simulink model "sf_fitness"  (R2017b)
settings: Solver=FixedStepAuto  StartTime=0.0  StopTime=inf  FixedStep=0.001  RelTol=1e-3  EnableMultiTasking=on
StopFcn:
  | close all force;
  | set_param('sf_fitness/Stop', 'Value', '0');
undefined symbols (not defined in the file): ActivityType
settings Model: Creator=The MathWorks, Inc.  LastModifiedBy=The MathWorks, Inc.
settings SolverCC: IsAutoAppliedInSIP=on
settings DataIOCC: LimitDataPoints=on
settings OptimizationCC: LifeSpan=inf
settings DebuggingCC: AllowSymbolicDim=off  SFUnexpectedBacktrackingDiag=warning  SFNoUnconditionalDefaultTransitionDiag=warning  SFExecutionAtInitializationDiag=none
settings ModelReferenceCC: PropagateSignalLabelsOutOfModel=off
settings CodeAppCC: StateflowObjectComments=on
settings GRTTargetCC: TargetLangStandard=C89/C90 (ANSI)
settings ConfigComp: CovMetricSettings=dw  CovHtmlReporting=on  CovSaveCumulativeToWorkspaceVar=on  CovSaveSingleToWorkspaceVar=on  CovExternalEMLEnable=off
settings SimscapeCC: SimscapeNormalizeSystem=off  SimscapeNominalValues={1, 'bar'; 1, 'cm^3/s'; 1, 'bar*kg/s'; 1, 'kJ/kg'; 1, 'kW'}

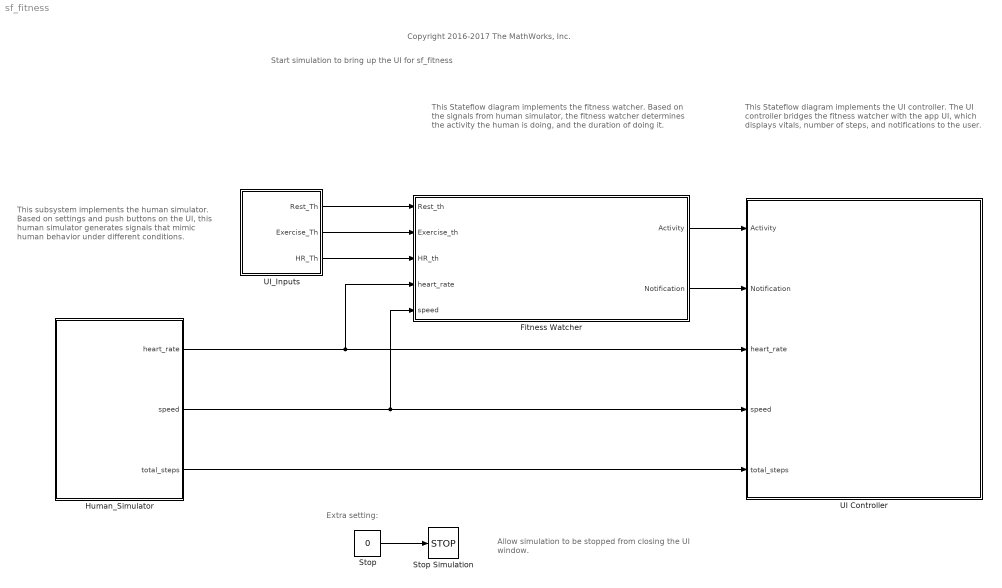
== system sf_fitness ==
  note: Extra setting:
  note: Allow simulation to be stopped from
      | closing the UI window.
  note: This subsystem implements
      | the human simulator.
      |
      | Based on settings and push buttons on
      | the UI, this human simulator generates
      | signals that mimic human behavior under
      | different conditions.
  note: This Stateflow diagram implements
      | the fitness watcher.
      |
      | Based on the signals from human simulator,
      | the fitness watcher determines the activity
      | the human is doing, and the duration of doing it.
  note: Start simulation to bring up the UI for sf_fitness
  note: This Stateflow diagram implements
      | the UI controller.
      |
      | The UI controller bridges the fitness watcher with the app UI, which displays vitals, number of steps, and notifications to the user.
  note: Copyright 2016-2017 The MathWorks, Inc.
  Fitness Watcher : Stateflow chart  TreatAsAtomicUnit=on
  Human_Simulator : Subsystem
  Stop : Constant  Value=0
  Stop Simulation : Stop
  UI Controller : Stateflow chart  TreatAsAtomicUnit=on
  UI_Inputs : Subsystem
  wires:
  Fitness Watcher/2(Notification) -> UI Controller/2(Notification)
  UI_Inputs/1(Rest_Th) -> Fitness Watcher/1(Rest_th)
  UI_Inputs/2(Exercise_Th) -> Fitness Watcher/2(Exercise_th)
  UI_Inputs/3(HR_Th) -> Fitness Watcher/3(HR_th)
  Fitness Watcher/1(Activity) -> UI Controller/1(Activity)
  Human_Simulator/1(heart_rate) -> Fitness Watcher/4(heart_rate), UI Controller/3(heart_rate)
  Human_Simulator/2(speed) -> Fitness Watcher/5(speed), UI Controller/4(speed)
  Human_Simulator/3(total_steps) -> UI Controller/5(total_steps)
  Stop/1 -> Stop Simulation/1

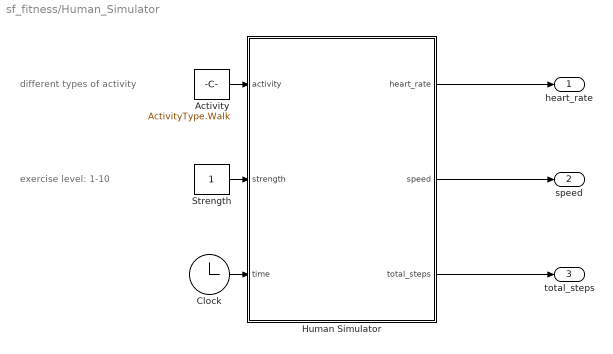
== system sf_fitness/Human_Simulator ==
  note: different types of activity
  note: exercise level: 1-10
  Activity : Constant  Value=ActivityType.Walk
  Clock : Clock
  Human Simulator : Stateflow chart  TreatAsAtomicUnit=on
  Strength : Constant
  heart_rate : Outport
  speed : Outport  Port=2
  total_steps : Outport  Port=3
  wires:
  Activity/1 -> Human Simulator/1(activity)
  Human Simulator/3(total_steps) -> total_steps/1
  Clock/1 -> Human Simulator/3(time)
  Strength/1 -> Human Simulator/2(strength)
  Human Simulator/1(heart_rate) -> heart_rate/1
  Human Simulator/2(speed) -> speed/1

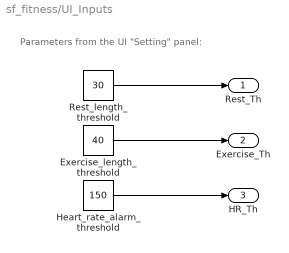
== system sf_fitness/UI_Inputs ==
  note: Parameters from the UI "Setting" panel:
  Exercise_length_threshold : Constant  Value=40
  Heart_rate_alarm_threshold : Constant  Value=150
  Rest_length_threshold : Constant  Value=30
  Rest_Th : Outport
  Exercise_Th : Outport  Port=2
  HR_Th : Outport  Port=3
  wires:
  Rest_length_threshold/1 -> Rest_Th/1
  Exercise_length_threshold/1 -> Exercise_Th/1
  Heart_rate_alarm_threshold/1 -> HR_Th/1

== stateflow chart sf_fitness/Human_Simulator/Human Simulator ==
  note: Units for variables:
      | speed: number of steps per second
      | heart_rate: beats per minute
  state Step_Tracker [parallel]
    en: total_steps = 0;
    settings: executionOrder=2
    state A
    state B
    (default) -> A
    A -> B : [after(1,sec)]{total_steps = total_steps + speed * 60;}
    B -> A
  state Simulator [parallel]
    en: heart_rate = 75; speed = 0;
    du:
    settings: executionOrder=1
    state Init
    state Sim_Sleep
      en: oldhr = heart_rate; olds = speed; oldt = time;
      du:
      [heart_rate, speed] = sim_sleep(oldhr, olds, time-oldt);
    state Sim_Rest
      en: oldhr = heart_rate; olds = speed; oldt = time;
      du:
      [heart_rate, speed] = sim_rest(oldhr,olds, time-oldt);
    state Sim_Walk
      en: oldhr = heart_rate; olds = speed; oldt = time;
      du:
      [heart_rate, speed] = sim_walk(oldhr, olds, time-oldt);
    state Sim_Exercise
      en: oldhr = heart_rate; olds = speed; oldt = time;
      du:
      [heart_rate, speed] = sim_exercise(oldhr,olds, time-oldt, strength);
    (default) -> Init
    Init -> (junction 257)
    (junction 257) -> Sim_Sleep [order 1] : [activity == ActivityType.Sleep]
    Sim_Sleep -> (junction 280)
    (junction 257) -> (junction 262) [order 2]
    (junction 280) -> (junction 281)
    Sim_Rest -> (junction 281)
    (junction 262) -> Sim_Rest [order 1] : [activity == ActivityType.Rest]
    (junction 281) -> (junction 282)
    (junction 262) -> (junction 264) [order 2]
    Sim_Walk -> (junction 282)
    (junction 264) -> Sim_Walk [order 1] : [activity == ActivityType.Walk]
    (junction 282) -> (junction 286)
    (junction 264) -> (junction 266) [order 2]
    (junction 266) -> Init [order 2]
    (junction 266) -> Sim_Exercise [order 1] : [activity == ActivityType.Exercise]
    Sim_Exercise -> (junction 286)
    (junction 286) -> (junction 287)
    (junction 288) -> Init
    (junction 287) -> (junction 288) : [hasChanged(activity)]
  data: old function_input; target function_input; result function_output; t function_input; oldHR function_input; oldS function_input; newTime function_input; heartRate function_output; Speed function_output; oldHR function_input; oldS function_input; newTime function_input; heartRate function_output; Speed function_output; oldHR function_input; oldS function_input; newTime function_input; heartRate function_output; Speed function_output; heartRate function_output; Speed function_output; oldHR function_input; oldS function_input; newTime function_input; Strength function_input; heart_rate output; speed output; activity input Enum: ActivityType; strength input; time input; oldhr local; olds local; oldt local; total_steps output
  function result = transition(old, target, t):
    | function result = transition(old, target, t)
    |     
    |     % use linear transition
    |     if t < 1 % all transition finish in 1 s; improve this later
    |         result = old + t * (target - old);
    |     else
    |         result = target;
    |     end
    |     
    | end
  function [heartRate, Speed] = sim_sleep(oldHR, oldS, newTime):
    | function [heartRate, Speed] = sim_sleep(oldHR, oldS, newTime)
    |    
    | target = 68;
    | 
    | % call transition function from oldHR to target
    | heartRate = transition(oldHR, target, newTime);
    | % update exercising speed
    | Speed = transition(oldS, 0, newTime);
    |     
    | end
  function [heartRate, Speed] = sim_rest(oldHR, oldS, newTime):
    | function [heartRate, Speed] = sim_rest(oldHR, oldS, newTime)
    |    
    | target = 75;
    | 
    | % call transition function from oldHR to target
    | heartRate = transition(oldHR, target, newTime);
    | % update exercising speed
    | Speed = transition(oldS, 0, newTime);
    |     
    | end
  function [heartRate, Speed] = sim_walk(oldHR, oldS, newTime):
    | function [heartRate, Speed] = sim_walk(oldHR, oldS, newTime)
    |    
    | target = 85;
    | 
    | % call transition function from oldHR to target
    | heartRate = transition(oldHR, target, newTime);
    | % update exercising speed
    | Speed = transition(oldS, 2, newTime);
    |     
    | end
  function [heartRate, Speed] = sim_exercise(oldHR, oldS, newTime, Strength):
    | function [heartRate, Speed] = sim_exercise(oldHR, oldS, newTime, Strength)
    | 
    | % strength is exercise level 1- 10
    | target = 85 + Strength * 8;
    | 
    | % call transition function from oldHR to target
    | heartRate = transition(oldHR, target, newTime);
    | % update exercising speed
    | % assume walk speed is 5
    | Speed = transition(oldS, (2 + 0.5 * Strength), newTime);
    | 
    | end

== stateflow chart sf_fitness/Fitness Watcher ==
  note: This chart has output activity monitoring child state activity, so the UI controller chart can display the detected activity.
      | Each state can send a Stateflow message, Notification, to the UI controller chart for notifications to be displayed such as Need_Exercise, Need_Rest etc.
      | Local data with initial value: sleep_heart_rate = 68 beats/minute; rest_heart_rate = 75 beats/minute; walk_speed = 2 steps/second.
  state Sleep
    exit:
    len = elapsed();
    sendNotification(len);
    state sendNotification(l) [function]
      (junction 410) -> (junction 413) : {Notification.data = sf_fitness_NotificationType.Sleep_Len; send(Notification);}
      (default) -> (junction 410) : [l>5]
  state Rest
    state Init
    state Send
      en:
      Notification.data = sf_fitness_NotificationType.Need_Exercise;
      send(Notification);
    (default) -> Rest.Init
    Rest.Init -> Rest.Send : [after(Rest_th, sec)]
  state Exercise
    state Timer [parallel]
      settings: executionOrder=1
      state Init
      state Send
        en:
        Notification.data = sf_fitness_NotificationType.Need_Rest;
        send(Notification);
      (default) -> Exercise.Timer.Init
      Exercise.Timer.Init -> Exercise.Timer.Send : [after(Exercise_th, sec)]
    state Exercise_Level [parallel]
      settings: executionOrder=2
      state Light_Exercise
      state Athlete
        state Init
        state Send
          en:
          Notification.data = sf_fitness_NotificationType.Slow_Down;
          send(Notification);
        (default) -> Exercise.Exercise_Level.Athlete.Init
        Exercise.Exercise_Level.Athlete.Init -> Exercise.Exercise_Level.Athlete.Send : after(15,sec)
      state Overheat
        state Init
        state Send
          en:
          Notification.data = sf_fitness_NotificationType.Must_Stop;
          send(Notification);
        (default) -> Exercise.Exercise_Level.Overheat.Init
        Exercise.Exercise_Level.Overheat.Init -> Exercise.Exercise_Level.Overheat.Send : [after(2,sec)]
      (default) -> Light_Exercise
      Light_Exercise -> Athlete : [speed > 4]
      Athlete -> Overheat [order 1] : [duration(heart_rate>HR_th) > 1]
      Overheat -> Athlete : [heart_rate < HR_th]
      Athlete -> Light_Exercise [order 2] : [speed < 4]
  state Walk
    exit:
    len = elapsed();
    sendNotification(len);
    state sendNotification(l) [function]
      (default) -> (junction 420) : [l>5]
      (junction 420) -> (junction 423) : {Notification.data = sf_fitness_NotificationType.Report_Steps; send(Notification);}
  (default) -> Rest
  (junction 320) -> Rest [order 1] : [speed < 0.01]
  Exercise -> (junction 320) : [duration(speed < walk_speed + 0.1)>2]
  Sleep -> Rest : [duration(heart_rate > rest_heart_rate-1)>2]
  (junction 320) -> (junction 317) [order 2]
  Rest -> Sleep [order 2] : [duration(heart_rate < sleep_heart_rate+1)>2]
  Rest -> (junction 317) [order 1] : [duration(speed > 0.01)>2]
  (junction 317) -> Exercise [order 1] : [speed > walk_speed + 0.1]
  (junction 317) -> Walk [order 2]
  Walk -> Rest [order 1] : [duration(speed < 0.01)>2]
  Walk -> Exercise [order 2] : [duration(speed > walk_speed+0.1)>2]
  data: l function_input double; l function_input double; Activity output Enum: ActivityType; Notification output Enum: sf_fitness_NotificationType; len local double; Rest_th input; Exercise_th input double; HR_th input double; heart_rate input double; speed input double; sleep_heart_rate local =68; rest_heart_rate local =75; walk_speed local =2

== stateflow chart sf_fitness/UI Controller ==
  state INIT [parallel]
    % Initialize Appdesigner app and import the App's interface.
    en:
    coder.extrinsic('sf_fitness_app', 'updateBeat', 'detectedActivity', 'updateSteps', 'updateClock', 'updateHeartRate', 'updateText');
    app = sf_fitness_app();
    settings: executionOrder=1
  state DISPLAY [parallel]
    % Update different displays on the user interface designed by Appdesigner
    settings: executionOrder=2
    state Activity [parallel]
      % Update detected activity
      settings: executionOrder=1
      state Idle
        en:steps = 0;
        du: time = elapsed();
      state SetActivity
        entry:
        detectedActivity(app, Activity);
      DISPLAY.Activity.Idle -> SetActivity : [hasChanged(Activity)]
      SetActivity -> DISPLAY.Activity.Idle
      (default) -> SetActivity
    state Steps [parallel]
      % Show stepping animation and total steps display
      settings: executionOrder=3
      state Still
      state Move
        en:
        state Idle
        state Update
          en: updateSteps(app, int32(total_steps));
        (default) -> DISPLAY.Steps.Move.Idle
        DISPLAY.Steps.Move.Update -> DISPLAY.Steps.Move.Idle
        DISPLAY.Steps.Move.Idle -> DISPLAY.Steps.Move.Update : [after(1,sec)]{steps = steps + 60*speed;}
      (default) -> Still
      Still -> Move : [speed > 0.01]
      Move -> Still : [speed < 0.01]
    state Vital [parallel]
      settings: executionOrder=4
      state Update
        en:
        % Update heart beat animation and
        % heart rate display
        interval = 60/heart_rate;
        updateBeat(app,interval/2);
        updateHeartRate(app, int32(heart_rate));
      (default) -> DISPLAY.Vital.Update
      DISPLAY.Vital.Update -> DISPLAY.Vital.Update : [after(interval,sec)]
    state Notification_and_Clock [parallel]
      settings: executionOrder=2
      state Clock
        % Keep clock going if no notification
        state Update
          en:
          updateClock(app, t);
        DISPLAY.Notification_and_Clock.Clock.Update -> DISPLAY.Notification_and_Clock.Clock.Update : after(1, sec)
      state Send_UI_Notification
        % Replace clock with notification for 5 seconds
        en:
        updateText(app, Notification.data, int32(time), int32(steps), t);
      (default) -> Clock
      Send_UI_Notification -> Clock : [after(5, sec) ]
      Clock -> Send_UI_Notification : Notification
  data: Activity input; Notification input; heart_rate input double; speed input double; total_steps input; steps local double; time local double; interval local double; app local ml
